simulink model "cav_adas_scenario1"  (R2022a)
settings: Solver=VariableStepAuto  StartTime=0.0  StopTime=200  MaxStep=1e-3  RelTol=1e-3
InitFcn:
  | % ****CHALLENGE CSAGV***** %
  | % ****CIRO ARENA P38/53***** %
  | clear
  | clc
  | close all
  | %% VEHICLE PARAMETERS
  | m   = 1521;  % 𝑣𝑒ℎ𝑖𝑐𝑙𝑒 𝑚𝑎𝑠𝑠
  | fr  = 0.015; % 𝑟𝑜𝑙𝑙𝑖𝑛𝑔 𝑟𝑒𝑠𝑖𝑠𝑡𝑎𝑛𝑐𝑒 𝑐𝑜𝑒𝑓𝑓𝑖𝑐𝑖𝑒𝑛𝑡
  | g   = 9.81;  % 𝑔𝑟𝑎𝑣𝑖𝑡𝑎𝑡𝑖𝑜𝑛𝑎𝑙 𝑎𝑐𝑐𝑒𝑙𝑒𝑟𝑎𝑡𝑖𝑜𝑛
  | rho = 1.2;   % 𝑎𝑖𝑟 𝑑𝑒𝑛𝑠𝑖𝑡𝑦
  | Cd  = 0.28;  % 𝑑𝑟𝑎𝑔 𝑐𝑜𝑒𝑓𝑓𝑖𝑐𝑖𝑒𝑛𝑡
  | Af  = 2.33;  % 𝑓𝑟𝑜𝑛𝑡𝑎𝑙 𝑎𝑟𝑒𝑎
  | eta = 0.93;  % 𝑡ℎ𝑒 𝑒𝑓𝑓𝑖𝑐𝑖𝑒𝑛𝑐𝑦
  | R   = 0.5;   % wheel radius
  | 
  | Kv = -1500;
  | Kp = -100;
  | d_default = 30;
  | Tgap = 10;
undefined symbols (not defined in the file or in its folder): M, sigbuilder_block
settings Model: Creator=user  LastModifiedBy=user

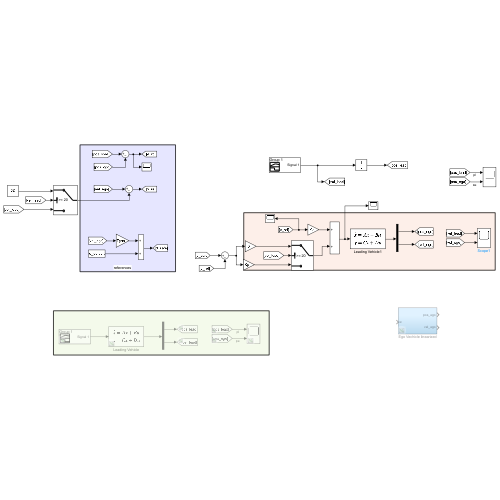
[thumbnail: Simulink's stored preview of the top-level diagram]
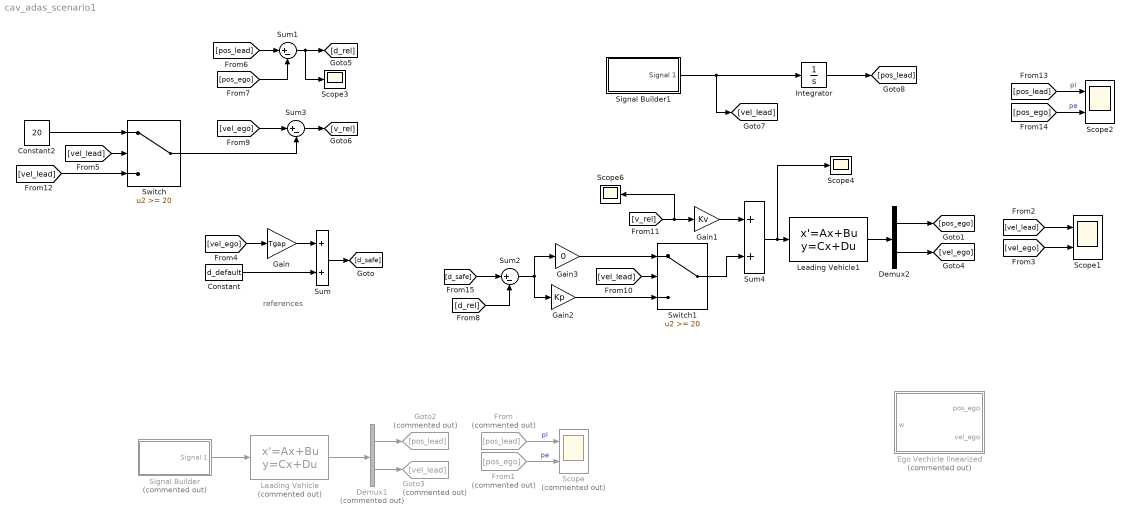
== system cav_adas_scenario1 ==
  note: references
  Constant : Constant  Value=d_default
  Constant2 : Constant  Value=20
  Demux1 : Demux  Commented=on  Outputs=2
  Demux2 : Demux  Outputs=2
  Ego Vechicle linearized : Subsystem  Commented=on
  From : From  Commented=on  GotoTag=pos_lead
  From1 : From  Commented=on  GotoTag=pos_ego
  Gain : Gain  Gain=Tgap
  Gain1 : Gain  Gain=Kv
  Gain2 : Gain  Gain=Kp
  Gain3 : Gain  Gain=0
  Goto2 : Goto  Commented=on  GotoTag=pos_lead
  Goto3 : Goto  Commented=on  GotoTag=vel_lead
  Integrator : Integrator  InitialCondition=200
  Leading Vehicle : StateSpace  Commented=on  A=[0 1; 0 0];  B=[0; 1];  C=eye(2)  D=[0; 0];  InitialCondition=[200, 20]
  Leading Vehicle1 : StateSpace  A=[0 1; 0 0];  B=[0; 1/m];  C=eye(2)  D=[0; 0];  InitialCondition=[150, 15]
  Scope : Scope  Commented=on  NumInputPorts=2
  Scope1 : Scope  NumInputPorts=2
  Scope2 : Scope  NumInputPorts=2
  Scope3 : Scope
  Scope4 : Scope
  Scope6 : Scope
  Signal Builder : Subsystem  Tag=STV Subsys  Commented=on  LoadFcn=sigbuilder_block('load');  StartFcn=sigbuilder_block('start');  StopFcn=sigbuilder_block('stop');  ClipboardFcn=sigbuilder_block('clipboard');  mask(Sigbuilder block){tuvar=[0:10]}
      mask help: Simulink:masks:SigbuilderBlock_MD
      mask init:
      | if ~strcmp(get_param(bdroot(gcbh),'SimulationStatus'),'stopped') tuvar = sigbuilder_block('maskInit'); end
      settings: CopyFcn=sigbuilder_block('copy');  DeleteFcn=sigbuilder_block('delete');  ModelCloseFcn=sigbuilder_block('modelClose');  PreSaveFcn=sigbuilder_block('preSave');  PauseFcn=sigbuilder_block('pause');  ContinueFcn=sigbuilder_block('continue');  NameChangeFcn=sigbuilder_block('namechange');  OpenFcn=sigbuilder_block('open',[391.2 97.2 550.8 400.2 ]);  CloseFcn=sigbuilder_block('close');
      mask Display: plot(0, 0, 100, 100,[2, 2, 32, 32, 2], [68, 8, 8, 68, 68],[32, 2], [38, 38], [32, 19, 2],[53, 60, 44], [32, 17, 17, 2],[16, 16, 31, 31]);txt = getActiveGroup(gcbh);text(2, 100, txt,'verticalAlignment', 'top');
  Signal Builder1 : Subsystem  Tag=STV Subsys  LoadFcn=sigbuilder_block('load');  StartFcn=sigbuilder_block('start');  StopFcn=sigbuilder_block('stop');  ClipboardFcn=sigbuilder_block('clipboard');  mask(Sigbuilder block){tuvar=[0:10]}
      mask help: Simulink:masks:SigbuilderBlock_MD
      mask init:
      | if ~strcmp(get_param(bdroot(gcbh),'SimulationStatus'),'stopped') tuvar = sigbuilder_block('maskInit'); end
      settings: CopyFcn=sigbuilder_block('copy');  DeleteFcn=sigbuilder_block('delete');  ModelCloseFcn=sigbuilder_block('modelClose');  PreSaveFcn=sigbuilder_block('preSave');  PauseFcn=sigbuilder_block('pause');  ContinueFcn=sigbuilder_block('continue');  NameChangeFcn=sigbuilder_block('namechange');  OpenFcn=sigbuilder_block('open',[391.2 97.2 550.8 400.2 ]);  CloseFcn=sigbuilder_block('close');
      mask Display: plot(0, 0, 100, 100,[2, 2, 32, 32, 2], [68, 8, 8, 68, 68],[32, 2], [38, 38], [32, 19, 2],[53, 60, 44], [32, 17, 17, 2],[16, 16, 31, 31]);txt = getActiveGroup(gcbh);text(2, 100, txt,'verticalAlignment', 'top');
  Sum : Sum
  Sum1 : Sum  Inputs=|+-
  Sum2 : Sum  Inputs=|+-
  Sum3 : Sum  Inputs=|+-
  Sum4 : Sum
  Switch : Switch  Threshold=20  SaturateOnIntegerOverflow=off  InputSameDT=off
  Switch1 : Switch  Threshold=20  SaturateOnIntegerOverflow=off  InputSameDT=off
  wires:
  Demux1/1 -> Goto2/1
  Leading Vehicle/1 -> Demux1/1
  Demux1/2 -> Goto3/1
  Demux2/1 -> [pos_ego]
  Demux2/2 -> [vel_ego]
  Signal Builder/1(Signal 1) -> Leading Vehicle/1
  From/1 -> Scope/1  "pl"
  From1/1 -> Scope/2  "pe"
  [vel_lead] -> Scope1/1
  [vel_ego] -> Scope1/2
  [vel_ego] -> Gain/1
  Gain/1 -> Sum/1
  Constant/1 -> Sum/2
  Sum/1 -> [d_safe]
  [pos_lead] -> Sum1/1
  [pos_ego] -> Sum1/2
  [d_safe] -> Sum2/1
  [d_rel] -> Sum2/2
  [vel_ego] -> Sum3/1
  Switch/1 -> Sum3/2
  Sum3/1 -> [v_rel]
  [v_rel] -> Scope6/1, Gain1/1
  Sum2/1 -> Gain3/1, Gain2/1
  Sum4/1 -> Scope4/1, Leading Vehicle1/1
  Gain1/1 -> Sum4/1
  Leading Vehicle1/1 -> Demux2/1
  [vel_lead] -> Switch/2
  Constant2/1 -> Switch/1
  [vel_lead] -> Switch/3
  [vel_lead] -> Switch1/2
  Gain2/1 -> Switch1/3
  Gain3/1 -> Switch1/1
  Switch1/1 -> Sum4/2
  Sum1/1 -> Scope3/1, [d_rel]
  Signal Builder1/1(Signal 1) -> [vel_lead], Integrator/1
  Integrator/1 -> [pos_lead]
  [pos_lead] -> Scope2/1  "pl"
  [pos_ego] -> Scope2/2  "pe"

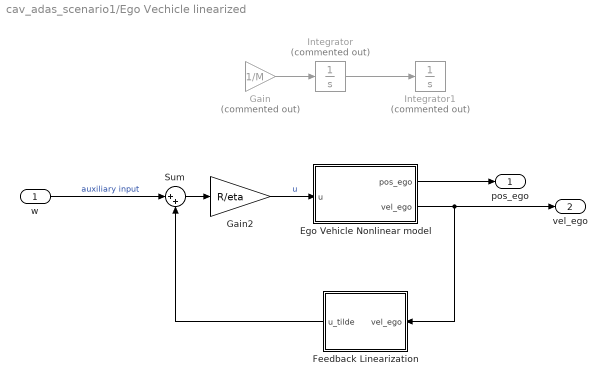
== system cav_adas_scenario1/Ego Vechicle linearized ==
  w : Inport
  Ego Vehicle Nonlinear model : Subsystem
  Feedback Linearization : Subsystem
  Gain : Gain  Commented=on  Gain=1/M
  Gain2 : Gain  Gain=R/eta
  Integrator : Integrator  Commented=on  InitialCondition=15
  Integrator1 : Integrator  Commented=on  InitialCondition=150
  Sum : Sum  Inputs=|++
  pos_ego : Outport
  vel_ego : Outport  Port=2
  wires:
  Gain/1 -> Integrator/1
  Integrator/1 -> Integrator1/1
  Ego Vehicle Nonlinear model/1(pos_ego) -> pos_ego/1
  Sum/1 -> Gain2/1
  Ego Vehicle Nonlinear model/2(vel_ego) -> vel_ego/1, Feedback Linearization/1(vel_ego)
  Feedback Linearization/1(u_tilde) -> Sum/2
  w/1 -> Sum/1  "auxiliary input"
  Gain2/1 -> Ego Vehicle Nonlinear model/1(u)  "u"

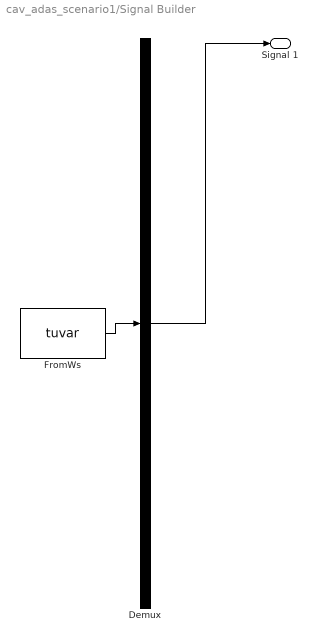
== system cav_adas_scenario1/Signal Builder ==
  Demux : Demux  Tag=STV Demux  Outputs=1
      settings: DisplayOption=none
  FromWs : FromWorkspace  Tag=STV FromWs  VariableName=tuvar
      SigBuilderData=|
      | common.afterFinalStr = 'Extrapolate'
      | common.sampleTime = 0
      | dataSet.timeRange = [0 200]
      | dataSet.name = 'Group 1'
      | sbobj.Groups.Name = 'Group 1'
      | sbobj.Groups.Signals.Name = 'Signal 1'
      | sbobj.Groups.Signals.XData = [0 40 40 80 80 120 120 200]
      | sbobj.Groups.Signals.YData = [1 1 0 0 -1 -1 0 0]
      | sbobj.Groups.TimeRange = [0 200]
  Signal 1 : Outport  Tag=STV Outport
  wires:
  Demux/1 -> Signal 1/1
  FromWs/1 -> Demux/1

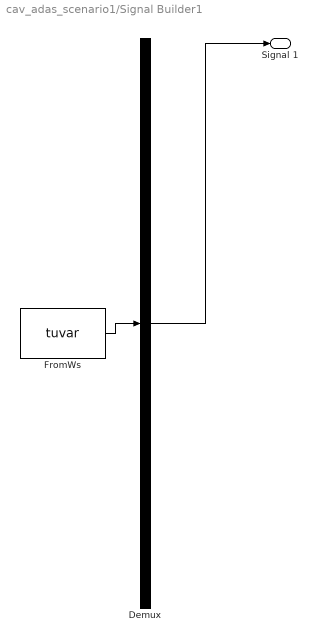
== system cav_adas_scenario1/Signal Builder1 ==
  Demux : Demux  Tag=STV Demux  Outputs=1
      settings: DisplayOption=none
  FromWs : FromWorkspace  Tag=STV FromWs  VariableName=tuvar
      SigBuilderData=|
      | common.afterFinalStr = 'Extrapolate'
      | common.sampleTime = 0
      | dataSet.timeRange = [0 200]
      | dataSet.name = 'Group 1'
      | sbobj.Groups.Name = 'Group 1'
      | sbobj.Groups.Signals.Name = 'Signal 1'
      | sbobj.Groups.Signals.XData = [0 40 40 90 90 140 140 200]
      | sbobj.Groups.Signals.YData = [20 20 10 10 30 30 0 0]
      | sbobj.Groups.TimeRange = [0 200]
  Signal 1 : Outport  Tag=STV Outport
  wires:
  FromWs/1 -> Demux/1
  Demux/1 -> Signal 1/1

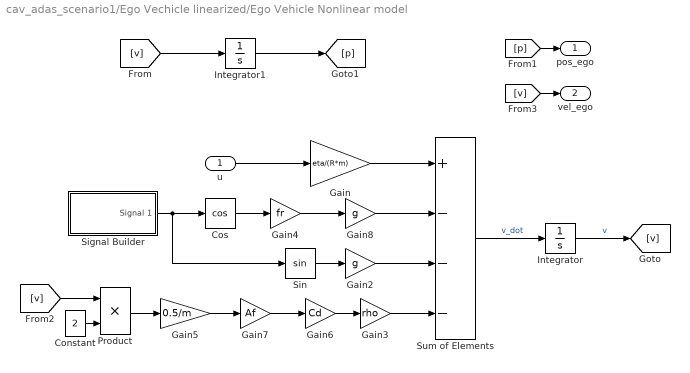
== system cav_adas_scenario1/Ego Vechicle linearized/Ego Vehicle Nonlinear model ==
  u : Inport
  Constant : Constant  Value=2
  Cos : Trigonometry  Operator=cos
  Gain : Gain  Gain=eta/(R*m)
  Gain2 : Gain  Gain=g
  Gain3 : Gain  Gain=rho
  Gain4 : Gain  Gain=fr
  Gain5 : Gain  Gain=0.5/m
  Gain6 : Gain  Gain=Cd
  Gain7 : Gain  Gain=Af
  Gain8 : Gain  Gain=g
  Integrator : Integrator
  Integrator1 : Integrator
  Product : Product
  Signal Builder : Subsystem  Tag=STV Subsys  LoadFcn=sigbuilder_block('load');  StartFcn=sigbuilder_block('start');  StopFcn=sigbuilder_block('stop');  ClipboardFcn=sigbuilder_block('clipboard');  mask(Sigbuilder block){tuvar=[0:10]}
      mask help: Simulink:masks:SigbuilderBlock_MD
      mask init:
      | if ~strcmp(get_param(bdroot(gcbh),'SimulationStatus'),'stopped') tuvar = sigbuilder_block('maskInit'); end
      settings: CopyFcn=sigbuilder_block('copy');  DeleteFcn=sigbuilder_block('delete');  ModelCloseFcn=sigbuilder_block('modelClose');  PreSaveFcn=sigbuilder_block('preSave');  PauseFcn=sigbuilder_block('pause');  ContinueFcn=sigbuilder_block('continue');  NameChangeFcn=sigbuilder_block('namechange');  OpenFcn=sigbuilder_block('open',[422.4 105 550.8 400.2 ]);  CloseFcn=sigbuilder_block('close');
      mask Display: plot(0, 0, 100, 100,[2, 2, 32, 32, 2], [68, 8, 8, 68, 68],[32, 2], [38, 38], [32, 19, 2],[53, 60, 44], [32, 17, 17, 2],[16, 16, 31, 31]);txt = getActiveGroup(gcbh);text(2, 100, txt,'verticalAlignment', 'top');
  Sin : Trigonometry
  Sum of Elements : Sum  Inputs=+---
  pos_ego : Outport
  vel_ego : Outport  Port=2
  wires:
  u/1 -> Gain/1
  Signal Builder/1(Signal 1) -> Sin/1, Cos/1
  Gain7/1 -> Gain6/1
  Sin/1 -> Gain2/1
  Gain8/1 -> Sum of Elements/2
  Product/1 -> Gain5/1
  Gain5/1 -> Gain7/1
  Gain3/1 -> Sum of Elements/4
  [p] -> pos_ego/1
  [v] -> Product/1
  [v] -> Integrator1/1
  Gain6/1 -> Gain3/1
  Integrator/1 -> [v]  "v"
  Integrator1/1 -> [p]
  Gain2/1 -> Sum of Elements/3
  Cos/1 -> Gain4/1
  Constant/1 -> Product/2
  Sum of Elements/1 -> Integrator/1  "v_dot"
  Gain4/1 -> Gain8/1
  Gain/1 -> Sum of Elements/1
  [v] -> vel_ego/1

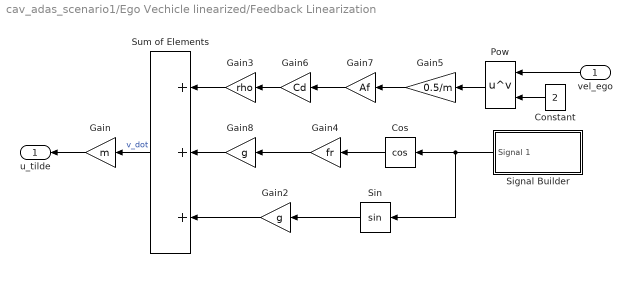
== system cav_adas_scenario1/Ego Vechicle linearized/Feedback Linearization ==
  vel_ego : Inport
  Constant : Constant  Value=2
  Cos : Trigonometry  Operator=cos
  Gain : Gain  Gain=m
  Gain2 : Gain  Gain=g
  Gain3 : Gain  Gain=rho
  Gain4 : Gain  Gain=fr
  Gain5 : Gain  Gain=0.5/m
  Gain6 : Gain  Gain=Cd
  Gain7 : Gain  Gain=Af
  Gain8 : Gain  Gain=g
  Pow : Math  Operator=pow  RndMeth=Zero
  Signal Builder : Subsystem  Tag=STV Subsys  LoadFcn=sigbuilder_block('load');  StartFcn=sigbuilder_block('start');  StopFcn=sigbuilder_block('stop');  ClipboardFcn=sigbuilder_block('clipboard');  mask(Sigbuilder block){tuvar=[0:10]}
      mask help: Simulink:masks:SigbuilderBlock_MD
      mask init:
      | if ~strcmp(get_param(bdroot(gcbh),'SimulationStatus'),'stopped') tuvar = sigbuilder_block('maskInit'); end
      settings: CopyFcn=sigbuilder_block('copy');  DeleteFcn=sigbuilder_block('delete');  ModelCloseFcn=sigbuilder_block('modelClose');  PreSaveFcn=sigbuilder_block('preSave');  PauseFcn=sigbuilder_block('pause');  ContinueFcn=sigbuilder_block('continue');  NameChangeFcn=sigbuilder_block('namechange');  OpenFcn=sigbuilder_block('open',[422.4 105 550.8 400.2 ]);  CloseFcn=sigbuilder_block('close');
      mask Display: plot(0, 0, 100, 100,[2, 2, 32, 32, 2], [68, 8, 8, 68, 68],[32, 2], [38, 38], [32, 19, 2],[53, 60, 44], [32, 17, 17, 2],[16, 16, 31, 31]);txt = getActiveGroup(gcbh);text(2, 100, txt,'verticalAlignment', 'top');
  Sin : Trigonometry
  Sum of Elements : Sum  Inputs=+++
  u_tilde : Outport
  wires:
  Pow/1 -> Gain5/1
  Gain3/1 -> Sum of Elements/1
  Gain7/1 -> Gain6/1
  vel_ego/1 -> Pow/1
  Sin/1 -> Gain2/1
  Signal Builder/1(Signal 1) -> Sin/1, Cos/1
  Gain8/1 -> Sum of Elements/2
  Constant/1 -> Pow/2
  Gain5/1 -> Gain7/1
  Gain6/1 -> Gain3/1
  Gain4/1 -> Gain8/1
  Gain2/1 -> Sum of Elements/3
  Cos/1 -> Gain4/1
  Sum of Elements/1 -> Gain/1  "v_dot"
  Gain/1 -> u_tilde/1

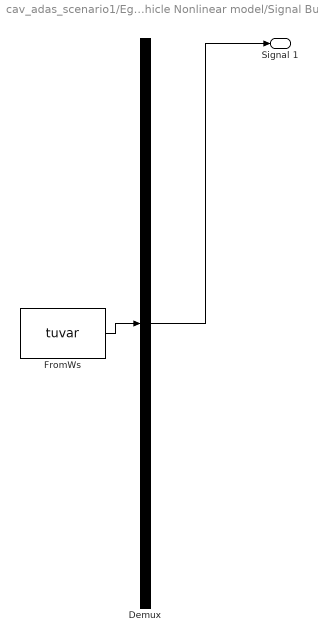
== system cav_adas_scenario1/Ego Vechicle linearized/Ego Vehicle Nonlinear model/Signal Builder ==
  Demux : Demux  Tag=STV Demux  Outputs=1
      settings: DisplayOption=none
  FromWs : FromWorkspace  Tag=STV FromWs  VariableName=tuvar
      SigBuilderData=|
      | common.afterFinalStr = 'Extrapolate'
      | common.sampleTime = 0
      | dataSet.timeRange = [0 10]
      | dataSet.name = 'Group 1'
      | sbobj.Groups.Name = 'Group 1'
      | sbobj.Groups.Signals.Name = 'Signal 1'
      | sbobj.Groups.Signals.XData = [0 3.33 3.33 6.66 6.66 10]
      | sbobj.Groups.Signals.YData = [-0.7854 -0.7854 0 0 0.7854 0.7854]
  Signal 1 : Outport  Tag=STV Outport
  wires:
  Demux/1 -> Signal 1/1
  FromWs/1 -> Demux/1

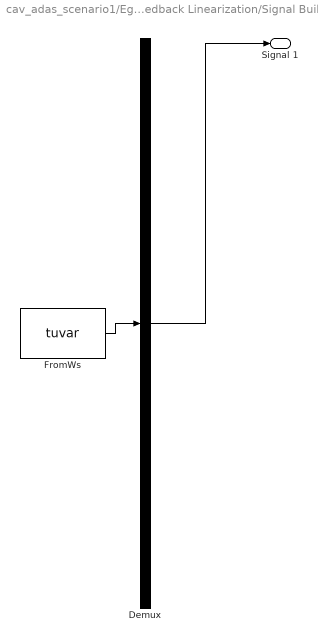
== system cav_adas_scenario1/Ego Vechicle linearized/Feedback Linearization/Signal Builder ==
  Demux : Demux  Tag=STV Demux  Outputs=1
      settings: DisplayOption=none
  FromWs : FromWorkspace  Tag=STV FromWs  VariableName=tuvar
      SigBuilderData=|
      | common.afterFinalStr = 'Extrapolate'
      | common.sampleTime = 0
      | dataSet.timeRange = [0 10]
      | dataSet.name = 'Group 1'
      | sbobj.Groups.Name = 'Group 1'
      | sbobj.Groups.Signals.Name = 'Signal 1'
      | sbobj.Groups.Signals.XData = [0 3.33 3.33 6.66 6.66 10]
      | sbobj.Groups.Signals.YData = [-0.7854 -0.7854 0 0 0.7854 0.7854]
  Signal 1 : Outport  Tag=STV Outport
  wires:
  Demux/1 -> Signal 1/1
  FromWs/1 -> Demux/1
